simulink model "pitch_axis_missile_IntegralControl_Simulink2022b"  (R2022b)
settings: Solver=ode4  StartTime=0.0  StopTime=SIM_TIME  FixedStep=STEP_SIZE  RelTol=1e-3
undefined symbols (not defined in the file): a_m, a_n, b_m, b_n, c_m, c_n, d_m, d_n, g, K_alpha, K_q, K_z, Kfs, Ki, M, StepAmplitude, Ts, uss, x0, xss, yss
settings Model: Creator=roga  LastModifiedBy=roga

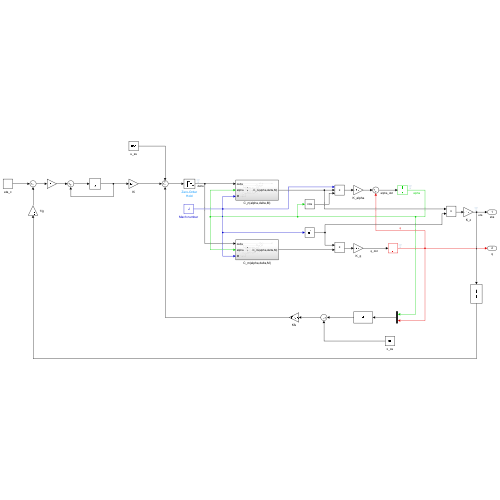
[thumbnail: Simulink's stored preview of the top-level diagram]
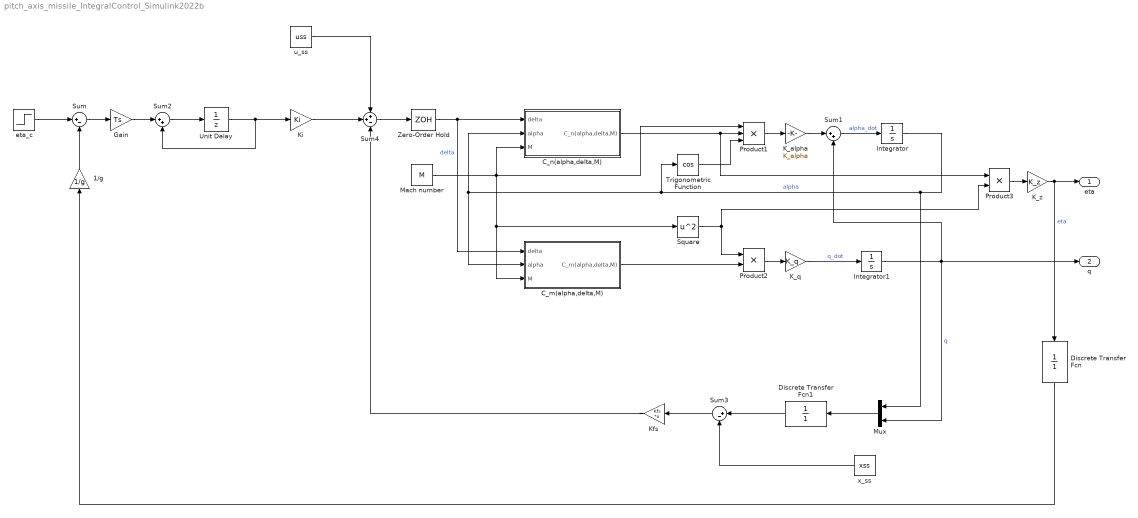
== system pitch_axis_missile_IntegralControl_Simulink2022b ==
  1/g : Gain  Gain=1/g
  C_m(alpha,delta,M) : Subsystem
  C_n(alpha,delta,M) : Subsystem
  Discrete Transfer Fcn : DiscreteTransferFcn  Denominator=[1]  SampleTime=Ts
  Discrete Transfer Fcn1 : DiscreteTransferFcn  Denominator=[1]  SampleTime=Ts
  Gain : Gain  Gain=Ts
  Integrator : Integrator  Priority=1  InitialCondition=x0(1)
  Integrator1 : Integrator  Priority=2  InitialCondition=x0(2)
  K_alpha : Gain  Gain=K_alpha
  K_q : Gain  Gain=K_q
  K_z : Gain  Gain=K_z
  Kfs : Gain  Gain=Kfs  Multiplication=Matrix(K*u) (u vector)
  Ki : Gain  Gain=Ki
  Mach number : Constant  Value=M
  Mux : Mux  Inputs=2
  Product1 : Product  Inputs=3
  Product2 : Product
  Product3 : Product
  Square : Math  Operator=square
  Sum : Sum  Inputs=|+-
  Sum1 : Sum  Inputs=|++
  Sum2 : Sum  Inputs=|++
  Sum3 : Sum  Inputs=|+-
  Sum4 : Sum  Inputs=++-
  Trigonometric Function : Trigonometry  Operator=cos
  Unit Delay : UnitDelay  SampleTime=Ts  HasFrameUpgradeWarning=on
  Zero-Order Hold : ZeroOrderHold  SampleTime=Ts
  eta_c : Step  Time=10  Before=yss(1)/g  After=yss(1)/g + StepAmplitude  SampleTime=Ts
  u_ss : Constant  Value=uss
  x_ss : Constant  Value=xss
  eta : Outport
  q : Outport  Port=2
  wires:
  Integrator1/1 -> Mux/2, q/1, Sum1/2  "q"
  Sum1/1 -> Integrator/1  "alpha_dot"
  K_alpha/1 -> Sum1/1
  Product1/1 -> K_alpha/1
  Trigonometric Function/1 -> Product1/3
  Integrator/1 -> Mux/1, C_m(alpha,delta,M)/2(alpha), C_n(alpha,delta,M)/2(alpha), Trigonometric Function/1  "alpha"
  Sum4/1 -> Zero-Order Hold/1
  C_n(alpha,delta,M)/1(C_n(alpha,delta,M)) -> Product1/2, Product3/1
  K_q/1 -> Integrator1/1  "q_dot"
  Product2/1 -> K_q/1
  Square/1 -> Product3/2, Product2/1
  C_m(alpha,delta,M)/1(C_m(alpha,delta,M)) -> Product2/2
  Mach number/1 -> C_m(alpha,delta,M)/3(M), Square/1, C_n(alpha,delta,M)/3(M), Product1/1
  K_z/1 -> eta/1, Discrete Transfer Fcn/1  "eta"
  Product3/1 -> K_z/1
  eta_c/1 -> Sum/1
  Sum/1 -> Gain/1
  Gain/1 -> Sum2/1
  Sum2/1 -> Unit Delay/1
  Unit Delay/1 -> Ki/1, Sum2/2
  1/g/1 -> Sum/2
  Mux/1 -> Discrete Transfer Fcn1/1
  Sum3/1 -> Kfs/1
  x_ss/1 -> Sum3/2
  Discrete Transfer Fcn/1 -> 1/g/1
  Ki/1 -> Sum4/2
  Kfs/1 -> Sum4/3
  u_ss/1 -> Sum4/1
  Zero-Order Hold/1 -> C_m(alpha,delta,M)/1(delta), C_n(alpha,delta,M)/1(delta)  "delta"
  Discrete Transfer Fcn1/1 -> Sum3/1

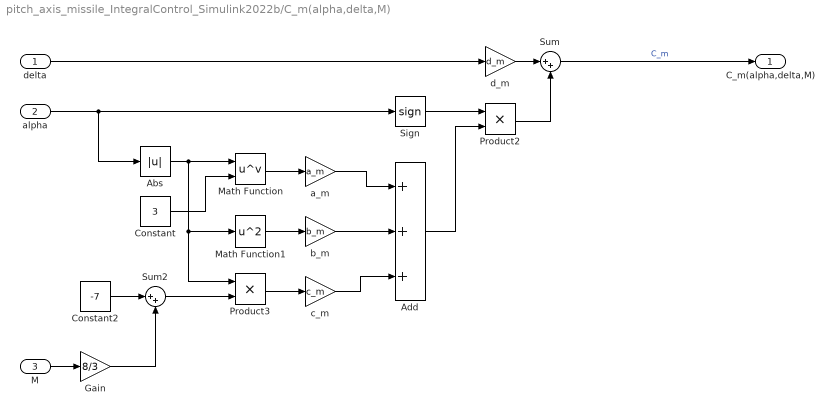
== system pitch_axis_missile_IntegralControl_Simulink2022b/C_m(alpha,delta,M) ==
  delta : Inport
  alpha : Inport  Port=2
  M : Inport  Port=3
  Abs : Abs  SaturateOnIntegerOverflow=off
  Add : Sum  Inputs=+++
  Constant : Constant  Value=3
  Constant2 : Constant  Value=-7
  Gain : Gain  Gain=8/3
  Math Function : Math  Operator=pow
  Math Function1 : Math  Operator=square
  Product2 : Product
  Product3 : Product
  Sign : Signum
  Sum : Sum  Inputs=|++
  Sum2 : Sum  Inputs=|++
  a_m : Gain  Gain=a_m
  b_m : Gain  Gain=b_m
  c_m : Gain  Gain=c_m
  d_m : Gain  Gain=d_m
  C_m(alpha,delta,M) : Outport
  wires:
  Gain/1 -> Sum2/2
  Sum/1 -> C_m(alpha,delta,M)/1  "C_m"
  Sum2/1 -> Product3/2
  Add/1 -> Product2/2
  Product2/1 -> Sum/2
  Constant/1 -> Math Function/2
  Math Function1/1 -> b_m/1
  b_m/1 -> Add/2
  Abs/1 -> Math Function/1, Math Function1/1, Product3/1
  alpha/1 -> Sign/1, Abs/1
  a_m/1 -> Add/1
  Product3/1 -> c_m/1
  d_m/1 -> Sum/1
  c_m/1 -> Add/3
  Constant2/1 -> Sum2/1
  Sign/1 -> Product2/1
  delta/1 -> d_m/1
  Math Function/1 -> a_m/1
  M/1 -> Gain/1

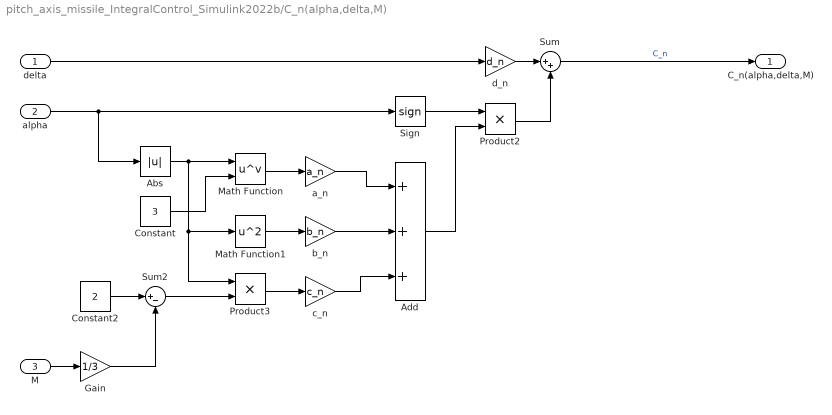
== system pitch_axis_missile_IntegralControl_Simulink2022b/C_n(alpha,delta,M) ==
  delta : Inport
  alpha : Inport  Port=2
  M : Inport  Port=3
  Abs : Abs  SaturateOnIntegerOverflow=off
  Add : Sum  Inputs=+++
  Constant : Constant  Value=3
  Constant2 : Constant  Value=2
  Gain : Gain  Gain=1/3
  Math Function : Math  Operator=pow
  Math Function1 : Math  Operator=square
  Product2 : Product
  Product3 : Product
  Sign : Signum
  Sum : Sum  Inputs=|++
  Sum2 : Sum  Inputs=|+-
  a_n : Gain  Gain=a_n
  b_n : Gain  Gain=b_n
  c_n : Gain  Gain=c_n
  d_n : Gain  Gain=d_n
  C_n(alpha,delta,M) : Outport
  wires:
  Math Function/1 -> a_n/1
  delta/1 -> d_n/1
  Sign/1 -> Product2/1
  Constant2/1 -> Sum2/1
  c_n/1 -> Add/3
  d_n/1 -> Sum/1
  Product3/1 -> c_n/1
  a_n/1 -> Add/1
  alpha/1 -> Abs/1, Sign/1
  Abs/1 -> Product3/1, Math Function1/1, Math Function/1
  b_n/1 -> Add/2
  Math Function1/1 -> b_n/1
  Constant/1 -> Math Function/2
  Product2/1 -> Sum/2
  Add/1 -> Product2/2
  Sum2/1 -> Product3/2
  Sum/1 -> C_n(alpha,delta,M)/1  "C_n"
  Gain/1 -> Sum2/2
  M/1 -> Gain/1
